simulink model "softstart_ramp_volt"  (R2019b)
settings: Solver=FixedStepAuto  StartTime=0.0  StopTime=5  FixedStep=Ts  RelTol=1e-3
values from neighbouring files (symbols this model uses):
  J = 0.25    [AM_4A225M2Y3.m]
  L1sig = x1sig/Wsn    [AM_4A225M2Y3.m]
  L2sig = x2sig/Wsn    [AM_4A225M2Y3.m]
  P2n = 55000    [AM_4A225M2Y3.m]
  r1 = tR1*Zb    [AM_4A225M2Y3.m]
  r2 = tR2*Zb    [AM_4A225M2Y3.m]
undefined symbols (not defined in the file or in its folder): f, ph_deg, Ts, Vm
libraries: powerlib x16
settings Model: Creator=NPT  LastModifiedBy=NPT

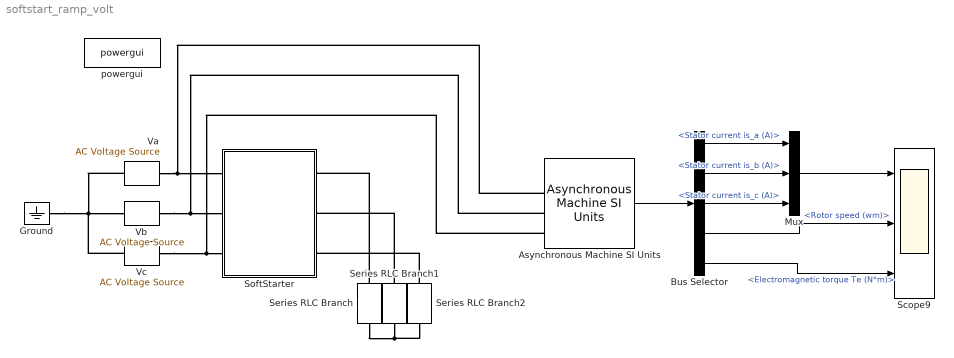
== system softstart_ramp_volt ==
  Asynchronous Machine SI Units : powerlib/Machines/Asynchronous Machine SI Units  RotorType=Squirrel-cage  PresetModel=No  MechanicalLoad=Torque Tm  ShowDetailedParameters=on  ReferenceFrame=Rotor  Units=SI  MeasurementBus=off  NominalParameters=[P2n 380 50]  Stator=[r1 L1sig]  Rotor=[r2 L2sig]  Cage1=[0.4155 0.002066]  Cage2=[0.4168 0.0003495]  Lm=L0  Mechanical=[J 0 1]  PolePairs=2  InitialConditions=[0 0 0 0 0 0 0 0]  SimulateSaturation=off  Saturation=[14.03593122, 27.81365428, 53.79336849, 72.68890987, 97.98006896, 148.6815601, 215.7428561, 302.9841135, 428.7778367 ; 230, 322, 414, 460, 506, 552, 598, 644, 690]  LoadFlowParameters=1492000  TsPowergui=0  TsBlock=-1  IterativeModel=Trapezoidal non iterative  IterativeDiscreteModel=Trapezoidal non iterative  Pmec=1.492e+006
      settings: SourceProductName=Simscape Electrical
  Bus Selector : BusSelector  OutputSignals=Stator measurements.Stator current is_a (A),Stator measurements.Stator current is_b (A),Stator measurements.Stator current is_c (A),Mechanical.Rotor speed (wm),Mechanical.Electromagnetic torque Te (N*m)
  Ground : powerlib/Elements/Ground  LConnTagsString=a
      settings: SourceProductName=Simscape Electrical
  Mux : Mux  Inputs=3
  Scope9 : Scope  NumInputPorts=3
  Series RLC Branch : powerlib/Elements/Series RLC Branch  LConnTagsString=__new0  RConnTagsString=__new0  BranchType=R  Resistance=100  Inductance=1e-3  SetiL0=off  InitialCurrent=0  Capacitance=1e-6  Setx0=off  InitialVoltage=0  Measurements=None
      settings: SourceProductName=Simscape Electrical
  Series RLC Branch1 : powerlib/Elements/Series RLC Branch  LConnTagsString=__new0  RConnTagsString=__new0  BranchType=R  Resistance=100  Inductance=1e-3  SetiL0=off  InitialCurrent=0  Capacitance=1e-6  Setx0=off  InitialVoltage=0  Measurements=None
      settings: SourceProductName=Simscape Electrical
  Series RLC Branch2 : powerlib/Elements/Series RLC Branch  LConnTagsString=__new0  RConnTagsString=__new0  BranchType=R  Resistance=100  Inductance=1e-3  SetiL0=off  InitialCurrent=0  Capacitance=1e-6  Setx0=off  InitialVoltage=0  Measurements=None
      settings: SourceProductName=Simscape Electrical
  SoftStarter : Subsystem
  Va : powerlib/Electrical Sources/AC Voltage Source  Amplitude=Vm  Phase=ph_deg(1)  Frequency=f  SampleTime=-1  Measurements=None  BusType=swing  Pref=10e3  Qref=0  Qmin=-inf  Qmax=+inf
      settings: SourceProductName=Simscape Electrical
  Vb : powerlib/Electrical Sources/AC Voltage Source  Amplitude=Vm  Phase=ph_deg(2)  Frequency=f  SampleTime=-1  Measurements=None  BusType=swing  Pref=10e3  Qref=0  Qmin=-inf  Qmax=+inf
      settings: SourceProductName=Simscape Electrical
  Vc : powerlib/Electrical Sources/AC Voltage Source  Amplitude=Vm  Phase=ph_deg(3)  Frequency=f  SampleTime=-1  Measurements=None  BusType=swing  Pref=10e3  Qref=0  Qmin=-inf  Qmax=+inf
      settings: SourceProductName=Simscape Electrical
  powergui : powerlib/powergui  Priority=1  SimulationMode=Discrete  SampleTime=Ts  frequency=60  Iterations=50  frequencyindice=50  Pbase=100e6  ErrMax=1e-4  UnitsV=kV  UnitsW=MW  buscounter=0  FunctionMessages=off  echomessages=off  EnableUseOfTLC=off  CurrentSourceSwitches=off  DisableSnubberDevices=off  DisableRonSwitches=off  DisableVfSwitches=off  DisplayEquations=off  AutomaticDiscreteSolvers=off  SolverType=Tustin  Interpol=off  ExternalGateDelay=off  methode=off  Ts=0  x0status=zero  SPID=off  SwTol=0  HookPort=off  NonlinearTolerance=1e-4  nMaxIteration=100  ContinueOnMaxIteration=off  RestoreLinks=warning  ResistiveCurrentMeasurement=off  Frange=[0:2:500]  Ylog=off  Xlog=on  ShowGrid=off  save=off  variable=ZData  structure=0  ZoomFFT=off  StartTime=0.0  cycles=1  DisplayStyle=1  fundamental=60  FreqAxis=off  MaxFrequency=1000  frequencyindicesteady=1  RmsSteady=1  display=off
      settings: SourceProductName=Simscape Electrical
  wires:
  Mux/1 -> Scope9/1
  Bus Selector/5 -> Scope9/3  "<Electromagnetic torque Te (N*m)>"
  Bus Selector/4 -> Scope9/2  "<Rotor speed (wm)>"
  Bus Selector/1 -> Mux/1  "<Stator current is_a (A)>"
  Bus Selector/2 -> Mux/2  "<Stator current is_b (A)>"
  Bus Selector/3 -> Mux/3  "<Stator current is_c (A)>"
  Asynchronous Machine SI Units/1 -> Bus Selector/1
  connections:
  Vc/LConn1 -- Ground/LConn1 -- Vb/LConn1 -- Va/LConn1
  Vb/RConn1 -- SoftStarter/LConn2 -- Asynchronous Machine SI Units/LConn2
  Va/RConn1 -- SoftStarter/LConn1 -- Asynchronous Machine SI Units/LConn1
  Vc/RConn1 -- Asynchronous Machine SI Units/LConn3 -- SoftStarter/LConn3
  Series RLC Branch/RConn1 -- Series RLC Branch2/RConn1 -- Series RLC Branch1/RConn1
  Series RLC Branch2/LConn1 -- SoftStarter/RConn3
  Series RLC Branch1/LConn1 -- SoftStarter/RConn2
  Series RLC Branch/LConn1 -- SoftStarter/RConn1

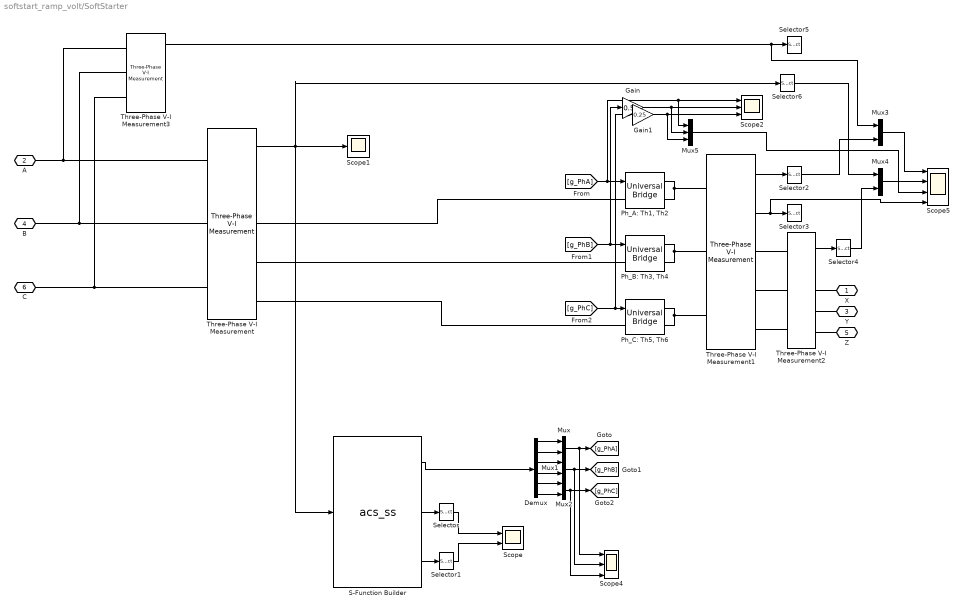
== system softstart_ramp_volt/SoftStarter ==
  Demux : Demux  Outputs=6
  Gain : Gain  Gain=0.5
  Gain1 : Gain  Gain=0.25
  Mux{,1..4} (5 alike) : Mux  Inputs=2
  Mux5 : Mux  Inputs=3
  "Ph_A: Th1, Th2" : powerlib/Power Electronics/Universal Bridge  Arms=1  SnubberResistance=1e5  SnubberCapacitance=inf  Device=Thyristors  Ron=1e-3  Lon=0  ForwardVoltages="[  0  0  ]"  ForwardVoltage=0  GTOparameters=[ 10e-6 , 20e-6 ]  IGBTparameters=[ 1e-6 , 2e-6 ]  Measurements=None  Measurements_2=None  converterType=Rectifier
      settings: SourceProductName=Simscape Electrical
  "Ph_B: Th3, Th4 " : powerlib/Power Electronics/Universal Bridge  Arms=1  SnubberResistance=1e5  SnubberCapacitance=inf  Device=Thyristors  Ron=1e-3  Lon=0  ForwardVoltages="[  0  0  ]"  ForwardVoltage=0  GTOparameters=[ 10e-6 , 20e-6 ]  IGBTparameters=[ 1e-6 , 2e-6 ]  Measurements=None  Measurements_2=None  converterType=Rectifier
      settings: SourceProductName=Simscape Electrical
  "Ph_C: Th5, Th6" : powerlib/Power Electronics/Universal Bridge  Arms=1  SnubberResistance=1e5  SnubberCapacitance=inf  Device=Thyristors  Ron=1e-3  Lon=0  ForwardVoltages="[  0  0  ]"  ForwardVoltage=0  GTOparameters=[ 10e-6 , 20e-6 ]  IGBTparameters=[ 1e-6 , 2e-6 ]  Measurements=None  Measurements_2=None  converterType=Rectifier
      settings: SourceProductName=Simscape Electrical
  S-Function Builder : S-Function  InitFcn=try, set_param(gcb,'FunctionName','acs_ss'), end  FunctionName=acs_ss  Parameters=100*Ts  SFunctionModules=acs_ss_wrapper integrator ss_file  SFunctionDeploymentMode=off  EnableBusSupport=off  mask(S-Function Builder){}
      mask help: Simulink:masks:SFunctionBuilder_MD
      mask init:
      | val = [[.9  0.75 0.75 1 1 .9 .9 1]',[1 1 0.75 0.75 .9 .9 1 .9]'];try , sys = get_param(gcb,'SfunBuilderFcnName');if isempty(sys), sys = get_param(gcb,'FunctionName'); end,catch, sys = get_param(gcb,'FunctionName'); end
      settings: CopyFcn=set_param(gcbh,'LinkStatus','none')  PreSaveFcn=try, set_param(gcb,'FunctionName','acs_ss'), end  OpenFcn=sfunctionwizard(gcbh)
      mask Display: plot(val(:,1),val(:,2)),disp(sys), port_label('input',1,'Vabc'), port_label('output',1,'gains'), port_label('output',2,'out'), port_label('output',3,'out2')
  Scope : Scope  NumInputPorts=2
  Scope1 : Scope
  Scope2 : Scope  NumInputPorts=3
  Scope4 : Scope  NumInputPorts=3
  Scope5 : Scope  NumInputPorts=4
  Selector : Selector  InputPortWidth=3  IndexOptions=Index vector (dialog)  Indices=[3]  OutputSizes=1
  Selector1 : Selector  InputPortWidth=3  IndexOptions=Index vector (dialog)  Indices=[3]  OutputSizes=1
  Selector{2..6} (5 alike) : Selector  InputPortWidth=3  IndexOptions=Index vector (dialog)  Indices=[1]  OutputSizes=1
  Three-Phase V-I Measurement : powerlib/Measurements/Three-Phase V-I Measurement  VoltageMeasurement=phase-to-phase  SetLabelV=off  LabelV=Vabc  Vpu=off  VpuLL=off  CurrentMeasurement=yes  SetLabelI=off  LabelI=Iabc  Ipu=off  Pbase=100e6  Vbase=500e3  OutputType=Complex  PhasorSimulation=off  PSBequivalent=0
      settings: SourceProductName=Simscape Electrical
  Three-Phase V-I Measurement1 : powerlib/Measurements/Three-Phase V-I Measurement  VoltageMeasurement=phase-to-ground  SetLabelV=off  LabelV=Vabc  Vpu=off  VpuLL=off  CurrentMeasurement=yes  SetLabelI=off  LabelI=Iabc  Ipu=off  Pbase=100e6  Vbase=500e3  OutputType=Complex  PhasorSimulation=off  PSBequivalent=0
      settings: SourceProductName=Simscape Electrical
  Three-Phase V-I Measurement2 : powerlib/Measurements/Three-Phase V-I Measurement  VoltageMeasurement=phase-to-phase  SetLabelV=off  LabelV=Vabc  Vpu=off  VpuLL=off  CurrentMeasurement=yes  SetLabelI=off  LabelI=Iabc  Ipu=off  Pbase=100e6  Vbase=500e3  OutputType=Complex  PhasorSimulation=off  PSBequivalent=0
      settings: SourceProductName=Simscape Electrical
  Three-Phase V-I Measurement3 : powerlib/Measurements/Three-Phase V-I Measurement  VoltageMeasurement=phase-to-ground  SetLabelV=off  LabelV=Vabc  Vpu=off  VpuLL=off  CurrentMeasurement=yes  SetLabelI=off  LabelI=Iabc  Ipu=off  Pbase=100e6  Vbase=500e3  OutputType=Complex  PhasorSimulation=off  PSBequivalent=0
      settings: SourceProductName=Simscape Electrical
  X : PMIOPort  Side=Right
  A : PMIOPort  Port=2  Side=Left
  Y : PMIOPort  Port=3  Side=Right
  B : PMIOPort  Port=4  Side=Left
  Z : PMIOPort  Port=5  Side=Right
  C : PMIOPort  Port=6  Side=Left
  wires:
  [g_PhA] -> Mux5/1, Scope2/1, "Ph_A: Th1, Th2"/1
  [g_PhB] -> "Ph_B: Th3, Th4 "/1, Gain/1
  [g_PhC] -> Gain1/1, "Ph_C: Th5, Th6"/1
  Three-Phase V-I Measurement/1 -> Selector6/1, S-Function Builder/1, Scope1/1
  Demux/1 -> Mux/1
  Demux/2 -> Mux/2
  Mux/1 -> Scope4/1, [g_PhA]
  Mux1/1 -> Scope4/2, [g_PhB]
  Demux/4 -> Mux1/2
  Demux/3 -> Mux1/1
  Demux/5 -> Mux2/1
  Demux/6 -> Mux2/2
  Mux2/1 -> Scope4/3, [g_PhC]
  S-Function Builder/1 -> Demux/1
  S-Function Builder/3 -> Selector1/1
  S-Function Builder/2 -> Selector/1
  Selector/1 -> Scope/1
  Selector1/1 -> Scope/2
  Three-Phase V-I Measurement1/1 -> Selector2/1
  Three-Phase V-I Measurement1/2 -> Scope5/4, Selector3/1
  Three-Phase V-I Measurement2/1 -> Selector4/1
  Selector2/1 -> Mux3/2
  Selector4/1 -> Mux4/2
  Three-Phase V-I Measurement3/1 -> Mux3/1, Selector5/1
  Mux3/1 -> Scope5/1
  Mux4/1 -> Scope5/2
  Selector6/1 -> Mux4/1
  Gain/1 -> Mux5/2, Scope2/2
  Gain1/1 -> Mux5/3, Scope2/3
  Mux5/1 -> Scope5/3
  connections:
  C/RConn1 -- Three-Phase V-I Measurement3/LConn3 -- Three-Phase V-I Measurement/LConn3
  B/RConn1 -- Three-Phase V-I Measurement3/LConn2 -- Three-Phase V-I Measurement/LConn2
  A/RConn1 -- Three-Phase V-I Measurement3/LConn1 -- Three-Phase V-I Measurement/LConn1
  Three-Phase V-I Measurement/RConn3 -- "Ph_C: Th5, Th6"/LConn1
  "Ph_A: Th1, Th2"/LConn1 -- Three-Phase V-I Measurement/RConn1
  "Ph_C: Th5, Th6"/RConn1 -- "Ph_C: Th5, Th6"/RConn2 -- Three-Phase V-I Measurement1/LConn3
  "Ph_B: Th3, Th4 "/RConn1 -- "Ph_B: Th3, Th4 "/RConn2 -- Three-Phase V-I Measurement1/LConn2
  "Ph_A: Th1, Th2"/RConn1 -- Three-Phase V-I Measurement1/LConn1 -- "Ph_A: Th1, Th2"/RConn2
  "Ph_B: Th3, Th4 "/LConn1 -- Three-Phase V-I Measurement/RConn2
  Three-Phase V-I Measurement1/RConn2 -- Three-Phase V-I Measurement2/LConn2
  Three-Phase V-I Measurement1/RConn1 -- Three-Phase V-I Measurement2/LConn1
  Three-Phase V-I Measurement1/RConn3 -- Three-Phase V-I Measurement2/LConn3
  Three-Phase V-I Measurement2/RConn1 -- X/RConn1
  Three-Phase V-I Measurement2/RConn2 -- Y/RConn1
  Three-Phase V-I Measurement2/RConn3 -- Z/RConn1
